simulink model "controllo_SS_no_obs2023bL_riscritto"  (R2023b)
settings: Solver=VariableStepAuto  StartTime=0.0  StopTime=1  RelTol=1e-3
values from neighbouring files (symbols this model uses):
  Ken_eta = Ken(:, n+1:end)    [LQ_KF_L.m]    (also in LQ_Luenberger_L.m = K(:, 4))
  Ken_x = Ken(:, 1:n)    [LQ_KF_L.m]    (also in LQ_Luenberger_L.m = K(:, 1:3))
undefined symbols (not defined in the file or in its folder): Lc, Rtot, x1_eq0, x2_eq0, x3_eq0
libraries: simulink x1
settings Model: Creator=Pronto all'uso  LastModifiedBy=lollo

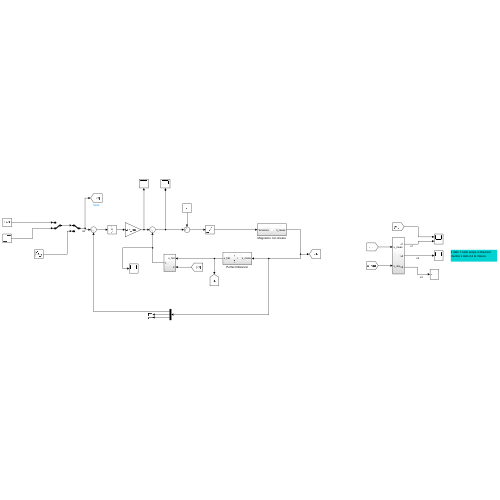
[thumbnail: Simulink's stored preview of the top-level diagram]
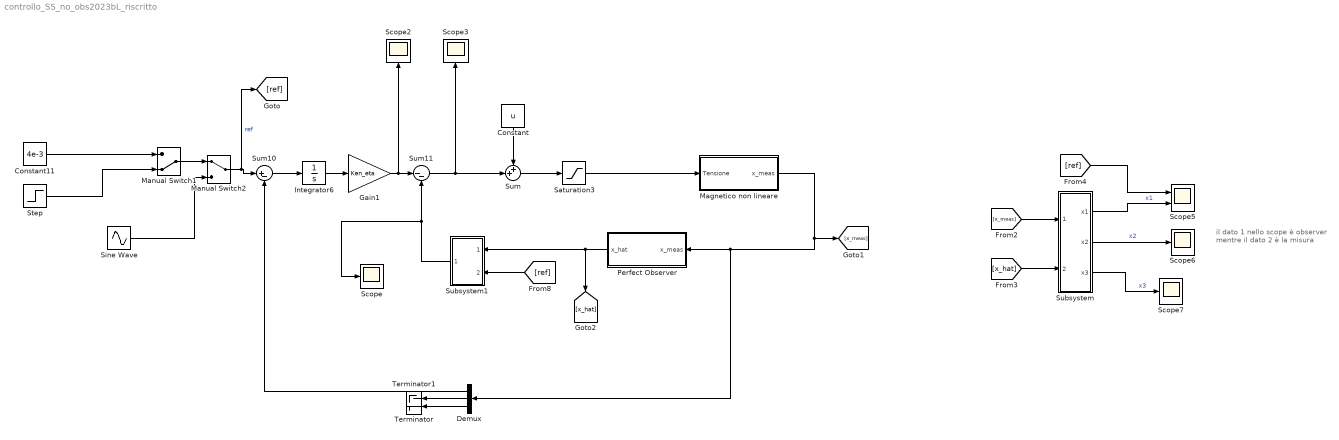
== system controllo_SS_no_obs2023bL_riscritto ==
  note: il dato 1 nello scope è observer
      | mentre il dato 2 è la misura
  Constant : Constant  Value=u
  Constant11 : Constant  Value=4e-3
  Demux : Demux  Outputs=3
  Gain1 : Gain  Gain=Ken_eta
  Integrator6 : Integrator
  Magnetico non lineare : Subsystem
  Manual Switch1 : ManualSwitch  CurrentSetting=0
  Manual Switch2 : ManualSwitch
  Perfect Observer : Subsystem
  Saturation3 : Saturate  UpperLimit=24  LowerLimit=-24
  Scope{,2..3,6..7} (5 alike) : Scope
  Scope5 : Scope  NumInputPorts=2
  Sine Wave : Sin  Amplitude=0.001  Bias=0.004  Frequency=4  SampleTime=0
  Step : Step  After=0.004  SampleTime=0
  Subsystem : Subsystem
  Subsystem1 : Subsystem
  Sum : Sum  Inputs=++|
  Sum10 : Sum  Inputs=|+-
  Sum11 : Sum  Inputs=|--
  Terminator : Terminator
  Terminator1 : Terminator
  wires:
  Sum11/1 -> Scope3/1, Sum/2
  Integrator6/1 -> Gain1/1
  Manual Switch1/1 -> Manual Switch2/1
  Sine Wave/1 -> Manual Switch2/2
  Manual Switch2/1 -> [ref], Sum10/1  "ref"
  Gain1/1 -> Sum11/1, Scope2/1
  Sum10/1 -> Integrator6/1
  Constant11/1 -> Manual Switch1/1
  Step/1 -> Manual Switch1/2
  Magnetico non lineare/1(x_meas) -> [x_meas], Demux/1, Perfect Observer/1(x_meas)
  Saturation3/1 -> Magnetico non lineare/1(Tensione)
  Demux/2 -> Terminator1/1
  Demux/3 -> Terminator/1
  Demux/1 -> Sum10/2
  Sum/1 -> Saturation3/1
  Constant/1 -> Sum/1
  [ref] -> Scope5/1
  Subsystem/1(x1) -> Scope5/2  "x1"
  Subsystem/3(x3) -> Scope7/1  "x3"
  [x_hat] -> Subsystem/2(x_obs)
  Subsystem/2(x2) -> Scope6/1  "x2"
  [x_meas] -> Subsystem/1(x_meas)
  [ref] -> Subsystem1/2(Input)
  Perfect Observer/1(x_hat) -> Subsystem1/1(x_hat), [x_hat]
  Subsystem1/1(Out1) -> Scope/1, Sum11/2

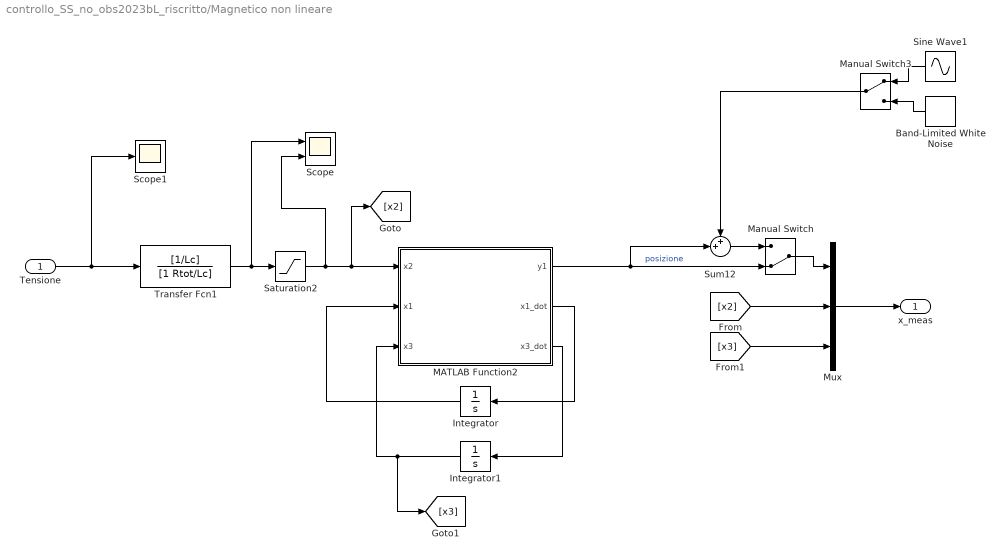
== system controllo_SS_no_obs2023bL_riscritto/Magnetico non lineare ==
  Tensione : Inport
  Band-Limited White Noise : simulink/Sources/Band-Limited White Noise  Cov=[8.9934e-11*0.002]  Ts=0.002  seed=[23341]
  Integrator : Integrator
  Integrator1 : Integrator
  MATLAB Function2 : MATLAB Function  TreatAsAtomicUnit=on
  Manual Switch : ManualSwitch  CurrentSetting=0
  Manual Switch3 : ManualSwitch
  Mux : Mux  Inputs=3
  Saturation2 : Saturate  UpperLimit=3  LowerLimit=0
  Scope : Scope  NumInputPorts=2
  Scope1 : Scope
  Sine Wave1 : Sin  Amplitude=0.00001  Frequency=50  SampleTime=0.002
  Sum12 : Sum  Inputs=++|
  Transfer Fcn1 : TransferFcn  Numerator=[1/Lc]  Denominator=[1 Rtot/Lc]
  x_meas : Outport
  wires:
  MATLAB Function2/1(y1) -> Manual Switch/2, Sum12/2  "posizione"
  MATLAB Function2/2(x1_dot) -> Integrator/1
  Integrator/1 -> MATLAB Function2/2(x1)
  MATLAB Function2/3(x3_dot) -> Integrator1/1
  Integrator1/1 -> [x3], MATLAB Function2/3(x3)
  Transfer Fcn1/1 -> Scope/1, Saturation2/1
  Saturation2/1 -> Scope/2, [x2], MATLAB Function2/1(x2)
  Tensione/1 -> Scope1/1, Transfer Fcn1/1
  [x2] -> Mux/2
  [x3] -> Mux/3
  Mux/1 -> x_meas/1
  Band-Limited White Noise/1 -> Manual Switch3/2
  Sine Wave1/1 -> Manual Switch3/1
  Manual Switch3/1 -> Sum12/1
  Sum12/1 -> Manual Switch/1
  Manual Switch/1 -> Mux/1

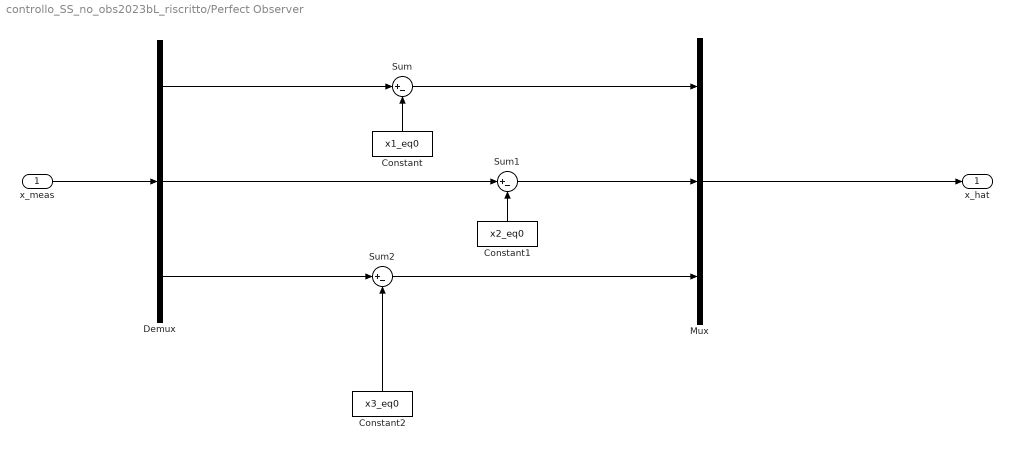
== system controllo_SS_no_obs2023bL_riscritto/Perfect Observer ==
  x_meas : Inport
  Constant : Constant  Value=x1_eq0
  Constant1 : Constant  Value=x2_eq0
  Constant2 : Constant  Value=x3_eq0
  Demux : Demux  Outputs=3
  Mux : Mux  Inputs=3
  Sum : Sum  Inputs=|+-
  Sum1 : Sum  Inputs=|+-
  Sum2 : Sum  Inputs=|+-
  x_hat : Outport
  wires:
  Demux/1 -> Sum/1
  Constant/1 -> Sum/2
  Constant1/1 -> Sum1/2
  Demux/2 -> Sum1/1
  Sum/1 -> Mux/1
  Sum1/1 -> Mux/2
  x_meas/1 -> Demux/1
  Demux/3 -> Sum2/1
  Mux/1 -> x_hat/1
  Constant2/1 -> Sum2/2
  Sum2/1 -> Mux/3

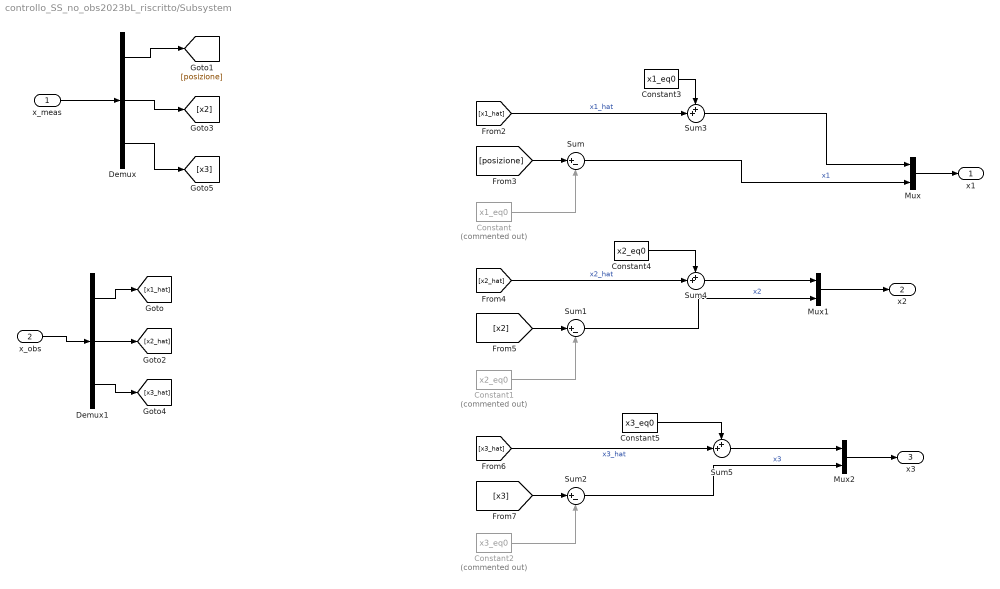
== system controllo_SS_no_obs2023bL_riscritto/Subsystem ==
  x_meas : Inport
  x_obs : Inport  Port=2
  Constant : Constant  Commented=on  Value=x1_eq0
  Constant1 : Constant  Commented=on  Value=x2_eq0
  Constant2 : Constant  Commented=on  Value=x3_eq0
  Constant3 : Constant  Value=x1_eq0
  Constant4 : Constant  Value=x2_eq0
  Constant5 : Constant  Value=x3_eq0
  Demux : Demux  Outputs=3
  Demux1 : Demux  Outputs=3
  Mux : Mux  Inputs=2
  Mux1 : Mux  Inputs=2
  Mux2 : Mux  Inputs=2
  Sum : Sum  Inputs=|+-
  Sum1 : Sum  Inputs=|+-
  Sum2 : Sum  Inputs=|+-
  Sum3 : Sum  Inputs=++|
  Sum4 : Sum  Inputs=++|
  Sum5 : Sum  Inputs=++|
  x1 : Outport
  x2 : Outport  Port=2
  x3 : Outport  Port=3
  wires:
  [posizione] -> Sum/1
  Constant1/1 -> Sum1/2
  Constant/1 -> Sum/2
  Sum1/1 -> Mux1/2  "x2"
  [x2] -> Sum1/1
  [x3] -> Sum2/1
  [x1_hat] -> Sum3/2  "x1_hat"
  Constant2/1 -> Sum2/2
  [x2_hat] -> Sum4/2  "x2_hat"
  [x3_hat] -> Sum5/2  "x3_hat"
  Sum2/1 -> Mux2/2  "x3"
  Sum/1 -> Mux/2  "x1"
  Demux/1 -> [posizione]
  Demux/2 -> [x2]
  Demux/3 -> [x3]
  Demux1/1 -> [x1_hat]
  Demux1/2 -> [x2_hat]
  Demux1/3 -> [x3_hat]
  x_obs/1 -> Demux1/1
  x_meas/1 -> Demux/1
  Mux/1 -> x1/1
  Mux1/1 -> x2/1
  Mux2/1 -> x3/1
  Sum3/1 -> Mux/1
  Sum4/1 -> Mux1/1
  Sum5/1 -> Mux2/1
  Constant3/1 -> Sum3/1
  Constant4/1 -> Sum4/1
  Constant5/1 -> Sum5/1

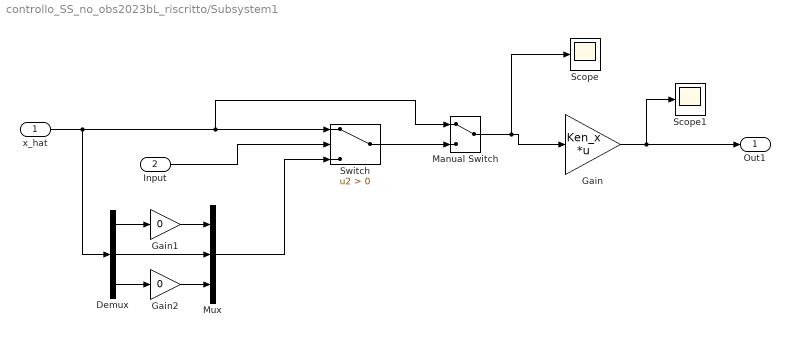
== system controllo_SS_no_obs2023bL_riscritto/Subsystem1 ==
  x_hat : Inport
  Input : Inport  Port=2
  Demux : Demux  Outputs=3
  Gain : Gain  Gain=Ken_x  Multiplication=Matrix(K*u) (u vector)
  Gain1 : Gain  Gain=0
  Gain2 : Gain  Gain=0
  Manual Switch : ManualSwitch
  Mux : Mux  Inputs=3
  Scope : Scope
  Scope1 : Scope
  Switch : Switch  Criteria=u2 > Threshold  SaturateOnIntegerOverflow=off  InputSameDT=off
  Out1 : Outport
  wires:
  Input/1 -> Switch/2
  Switch/1 -> Manual Switch/2
  x_hat/1 -> Demux/1, Manual Switch/1, Switch/1
  Gain/1 -> Scope1/1, Out1/1
  Manual Switch/1 -> Scope/1, Gain/1
  Demux/2 -> Mux/2
  Gain1/1 -> Mux/1
  Demux/1 -> Gain1/1
  Demux/3 -> Gain2/1
  Gain2/1 -> Mux/3
  Mux/1 -> Switch/3

== matlab function controllo_SS_no_obs2023bL_riscritto/Magnetico non lineare/MATLAB Function2 ==
  data: y1 output; x2 input; x1_dot output; x1 input; x3 input; x3_dot output
function [y1,x1_dot, x3_dot] = fcn(x2, x1, x3)
    m = 0.0657;
    g = 9.81;
    k_mag = 2.4405e-05;
    Rtot = 9.7585;
    Lc = 0.3708;
    y0 = 0.012;
    
    x1_dot = x3;
    if x1 < y0
        x3_dot = (k_mag/m)*(x2/(y0-x1))^2 - g;
    else
        x1 = 0.012;
        x3_dot = 0;
        x3 = 0;
    end

    
    % condizioni
    if x1 <=0 && x3_dot < 0
        x1 = 0;
        x3 = 0;
        x3_dot = 0;
    end
y1 = x1;
